simulink model "sim_main_esb_13"  (R2018b)
settings: Solver=VariableStepAuto  StartTime=0.0  StopTime=10.0  RelTol=1e-3
values from neighbouring files (symbols this model uses):
  A_klm = A_sys    [main_tf_12.m]    (also in main_tf_13.m = A_sys(1:6 , 1:6))
  A_sys = A    [main_tf_12.m]    (also in main_tf_13.m)
  B_klm = B_sys    [main_tf_12.m]    (also in main_tf_13.m = B_sys(1:6 , :))
  B_sys = B    [main_tf_12.m]    (also in main_tf_13.m)
  C = 0.344    [KALMAN.m]    (also in main_sys.m = double( subs( C) ); main_sys_klm.m = double( subs( C) ); main_tf_0.m = [ 0 , 0  , Ks , ds , -Ks , -ds, 0 ]; main_tf_1.m = C_mes)
  C_klm = C_sys    [main_tf_12.m]    (also in main_tf_13.m = C_sys(: , 1:6 ))
  C_sys_mod = eye(7,7)    [main_tf_12.m]    (also in main_tf_13.m)
  Ct = double( subs( Ct) )    [main_sys.m]    (also in main_sys_klm.m; main_tf_10.m; main_tf_11.m; main_tf_12.m)
  D_klm = D_sys    [main_tf_12.m]    (also in main_tf_13.m)
  D_sys_mod = zeros(7,2)    [main_tf_12.m]    (also in main_tf_13.m)
  Rk = 1    [main_sys_klm.m]    (also in main_tf_10.m; main_tf_11.m; main_tf_12.m = diag([ 10e-8 , 2.25e-8]); main_tf_13.m = diag([ 10e-8 , 2.25e-8]))
  Trq_mot_nom = .56    (= 0.56)    [main_cntl.m]    (also in main_sys.m; main_sys_klm.m; main_tf_10.m; main_tf_11.m)
  Tsk = .001    (= 0.001)    [main_tf_11.m]    (also in main_tf_12.m; main_tf_13.m)
  v_trq = 35e-3    (= 0.035)    [main_tf_11.m]    (also in main_tf_12.m; main_tf_13.m)
  v_vel = .1e-6    (= 1e-07)    [main_tf_11.m]    (also in main_tf_12.m; main_tf_13.m)
  w_trq = .1e-3    (= 0.0001)    [main_tf_11.m]    (also in main_tf_12.m; main_tf_13.m)
  w_vel = .15e-3    (= 0.00015)    [main_tf_11.m]    (also in main_tf_12.m; main_tf_13.m)
undefined symbols (not defined in the file or in its folder): Continuous, K_lq, K_lq3, Time
libraries: ctrlSharedLib x1
settings Model: Creator=eshojaei  LastModifiedBy=eshojaei

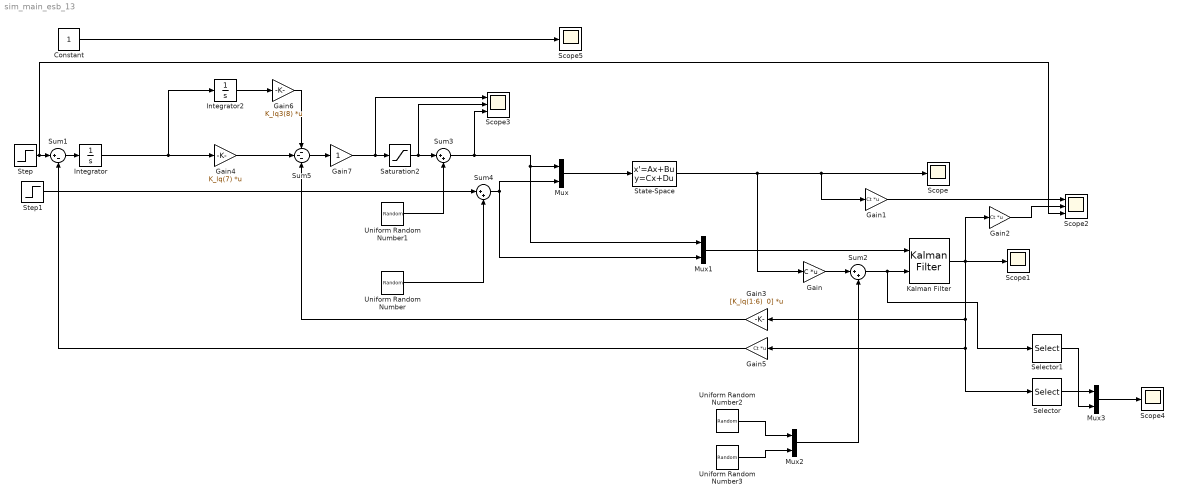
== system sim_main_esb_13 ==
  Constant : Constant
  Gain : Gain  Gain=C  Multiplication=Matrix(K*u)
  Gain1 : Gain  Gain=Ct  Multiplication=Matrix(K*u)
  Gain2 : Gain  Gain=Ct  Multiplication=Matrix(K*u)
  Gain3 : Gain  Gain="[K_lq(1:6)  0]"  Multiplication=Matrix(K*u)
  Gain4 : Gain  Gain=K_lq(7)  Multiplication=Matrix(K*u)
  Gain5 : Gain  Gain=Ct  Multiplication=Matrix(K*u)
  Gain6 : Gain  Gain=K_lq3(8)  Multiplication=Matrix(K*u)
  Gain7 : Gain
  Integrator : Integrator
  Integrator2 : Integrator
  Kalman Filter : ctrlSharedLib/Kalman Filter  TimeDomain=Continuous-Time  UseCurrentEstimator=on  ModelSource=Individual A, B, C, D matrices  ModelSourceVariable=ss(0.95,1,1,0,1)  A=A_klm  B=B_klm  C=C_klm  D=D_klm  NumberOfStates=1  NumberOfInputs=1  NumberOfOutputs=1  InitialEstimateSource=Dialog  X0=0  P0=10  UseK=off  UseGH=off  NumberOfProcessNoiseInputs=1  G=1  TimeInvariantG=on  H=0  TimeInvariantH=on  Q=Qk  TimeInvariantQ=on  R=Rk  TimeInvariantR=on  N=0  TimeInvariantN=on  AddInputPort=on  AddEnablePort=off  OutputEstimatedY=off  OutputP=off  Ts=-1
      settings: SourceProductBaseCode=CT
  Mux{,1..3} (4 alike) : Mux  Inputs=2
  Saturation2 : Saturate  UpperLimit=Trq_mot_nom  LowerLimit=-Trq_mot_nom
  Scope{,1,4..5} (4 alike) : Scope
  Scope2 : Scope  NumInputPorts=3
  Scope3 : Scope  NumInputPorts=3
  Selector : Selector  InputPortWidth=7  IndexOptions=Index vector (dialog)  Indices=[2]  OutputSizes=1
  Selector1 : Selector  InputPortWidth=2  IndexOptions=Index vector (dialog)  Indices=[1]  OutputSizes=1
  State-Space : StateSpace  A=A_sys  B=B_sys  C=C_sys_mod  D=D_sys_mod  InitialCondition=0
  Step : Step  Time=.1  After=5  SampleTime=0
  Step1 : Step  Time=.1  After=-.02  SampleTime=0
  Sum1 : Sum  Inputs=|+-
  Sum2 : Sum  Inputs=|++
  Sum3 : Sum  Inputs=|++
  Sum4 : Sum  Inputs=|++
  Sum5 : Sum  Inputs=---
  Uniform Random Number : UniformRandomNumber  Minimum=-w_vel  Maximum=w_vel  Seed=1  SampleTime=Tsk
  Uniform Random Number1 : UniformRandomNumber  Minimum=-w_trq  Maximum=w_trq  SampleTime=Tsk
  Uniform Random Number2 : UniformRandomNumber  Minimum=-v_vel  Maximum=v_vel  SampleTime=Tsk
  Uniform Random Number3 : UniformRandomNumber  Minimum=-v_trq  Maximum=v_trq  SampleTime=Tsk
  wires:
  Mux/1 -> State-Space/1
  State-Space/1 -> Gain/1, Gain1/1, Scope/1
  Step1/1 -> Sum4/1
  Kalman Filter/1 -> Selector/1, Gain5/1, Gain3/1, Gain2/1, Scope1/1
  Mux1/1 -> Kalman Filter/1
  Gain1/1 -> Scope2/1
  Gain2/1 -> Scope2/2
  Gain3/1 -> Sum5/3
  Sum5/1 -> Gain7/1
  Gain4/1 -> Sum5/2
  Step/1 -> Scope2/3, Sum1/1
  Sum1/1 -> Integrator/1
  Gain5/1 -> Sum1/2
  Uniform Random Number2/1 -> Mux2/1
  Uniform Random Number3/1 -> Mux2/2
  Gain/1 -> Sum2/1
  Sum2/1 -> Selector1/1, Kalman Filter/2
  Mux2/1 -> Sum2/2
  Saturation2/1 -> Scope3/2, Sum3/1
  Uniform Random Number1/1 -> Sum3/2
  Sum4/1 -> Mux/2, Mux1/2
  Uniform Random Number/1 -> Sum4/2
  Selector/1 -> Mux3/1
  Selector1/1 -> Mux3/2
  Mux3/1 -> Scope4/1
  Integrator2/1 -> Gain6/1
  Integrator/1 -> Gain4/1, Integrator2/1
  Gain6/1 -> Sum5/1
  Sum3/1 -> Mux/1, Mux1/1, Scope3/3
  Gain7/1 -> Scope3/1, Saturation2/1
  Constant/1 -> Scope5/1
